simulink model "TP4_1"  (R2016a)
settings: Solver=VariableStepAuto  StartTime=0.0  StopTime=4*pi*sqrt(10/9.81)  FixedStep=4*pi*sqrt(10/9.81) / 500  RelTol=1e-6
undefined symbols (not defined in the file): DiscIntNeverNeededParam, sigbuilder_block
libraries: simulink x5
settings Model: Creator=nsurbayr  LastModifiedBy=nsurbayr
settings DebuggingCC: MultiTaskRateTransMsg=warning

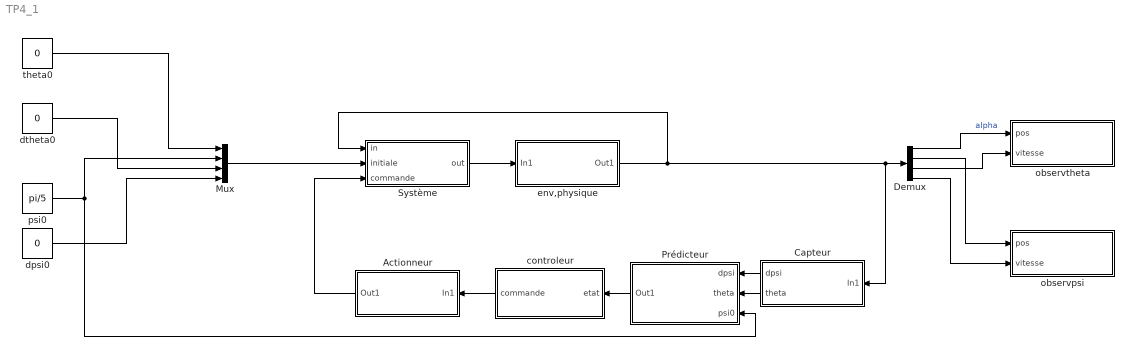
== system TP4_1 ==
  Actionneur : Subsystem
  Capteur : Subsystem
  Demux : Demux
  Mux : Mux
  Prédicteur : Subsystem
  Système : Subsystem
  controleur : Subsystem
  dpsi0 : Constant  Value=0  VectorParams1D=off
  dtheta0 : Constant  Value=0  VectorParams1D=off
  env,physique : Subsystem
  observpsi : Subsystem
  observtheta : Subsystem
  psi0 : Constant  Value=pi/5  VectorParams1D=off
  theta0 : Constant  Value=0
  wires:
  Système/1(out) -> env,physique/1(In1)
  controleur/1(commande) -> Actionneur/1(In1)
  Actionneur/1(Out1) -> Système/3(commande)
  env,physique/1(Out1) -> Système/1(in), Capteur/1(In1), Demux/1
  Prédicteur/1(Out1) -> controleur/1(etat)
  Capteur/1(dpsi) -> Prédicteur/1(dpsi)
  theta0/1 -> Mux/1
  Mux/1 -> Système/2(initiale)
  psi0/1 -> Prédicteur/3("psi0 "), Mux/2
  dtheta0/1 -> Mux/3
  dpsi0/1 -> Mux/4
  Demux/1 -> observtheta/1(pos)  "alpha"
  Demux/2 -> observpsi/1(pos)
  Demux/3 -> observtheta/2(vitesse)
  Demux/4 -> observpsi/2(vitesse)
  Capteur/2(theta) -> Prédicteur/2(theta)

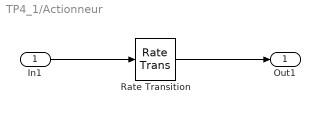
== system TP4_1/Actionneur ==
  In1 : Inport
  Rate Transition : RateTransition  X0=-1
  Out1 : Outport
  wires:
  Rate Transition/1 -> Out1/1
  In1/1 -> Rate Transition/1

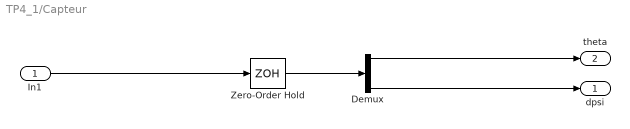
== system TP4_1/Capteur ==
  In1 : Inport
  Demux : Demux
  Zero-Order Hold : ZeroOrderHold  SampleTime=0.003
  dpsi : Outport
  theta : Outport  Port=2
  wires:
  In1/1 -> Zero-Order Hold/1
  Zero-Order Hold/1 -> Demux/1
  Demux/4 -> dpsi/1
  Demux/1 -> theta/1

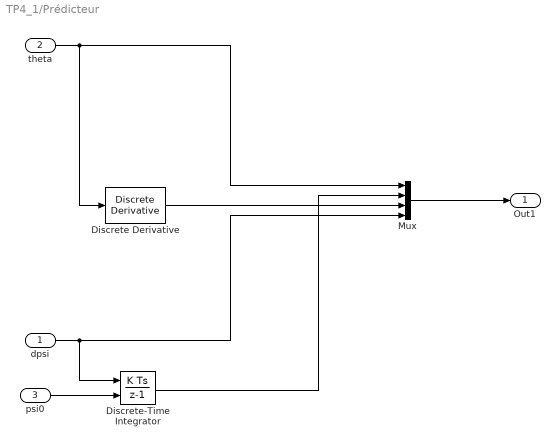
== system TP4_1/Prédicteur ==
  dpsi : Inport
  theta : Inport  Port=2
  "psi0 " : Inport  Port=3
  Discrete Derivative : simulink/Discrete/Discrete Derivative  gainval=1.0  ICPrevScaledInput=0.0  OutMin=[]  OutMax=[]  OutDataType=fixdt(1, 16)  OutScaling=2^-10  DoSatur=off
  Discrete-Time Integrator : DiscreteIntegrator  InitialConditionSource=external  InitialConditionSetting=State (most efficient)  SampleTime=-1  ICPrevOutput=DiscIntNeverNeededParam  ICPrevScaledInput=DiscIntNeverNeededParam
  Mux : Mux
  Out1 : Outport
  wires:
  Mux/1 -> Out1/1
  theta/1 -> Discrete Derivative/1, Mux/1
  dpsi/1 -> Discrete-Time Integrator/1, Mux/4
  Discrete Derivative/1 -> Mux/3
  "psi0 "/1 -> Discrete-Time Integrator/2
  Discrete-Time Integrator/1 -> Mux/2

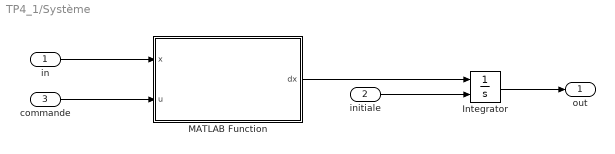
== system TP4_1/Système ==
  in : Inport
  initiale : Inport  Port=2
  commande : Inport  Port=3
  Integrator : Integrator  InitialConditionSource=external
  MATLAB Function : MATLAB Function  TreatAsAtomicUnit=on
      settings: RTWSystemCode=Inline
  out : Outport
  wires:
  Integrator/1 -> out/1
  initiale/1 -> Integrator/2
  in/1 -> MATLAB Function/1(x)
  commande/1 -> MATLAB Function/2(u)
  MATLAB Function/1(dx) -> Integrator/1

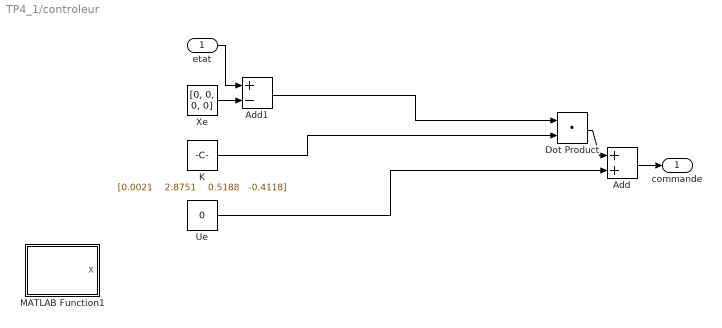
== system TP4_1/controleur ==
  etat : Inport
  Add : Sum
  Add1 : Sum  Inputs=+-
  Dot Product : DotProduct  InputSameDT=on  OutDataTypeStr=Inherit: Inherit via internal rule
  K : Constant  Value="[0.0021    2.8751    0.5188   -0.4118]"
  MATLAB Function1 : MATLAB Function  TreatAsAtomicUnit=on
  Ue : Constant  Value=0
  Xe : Constant  Value=[0, 0, 0, 0]
  commande : Outport
  wires:
  Add/1 -> commande/1
  Ue/1 -> Add/2
  Dot Product/1 -> Add/1
  K/1 -> Dot Product/2
  Xe/1 -> Add1/2
  etat/1 -> Add1/1
  Add1/1 -> Dot Product/1

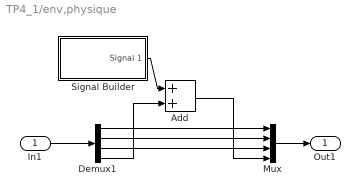
== system TP4_1/env,physique ==
  In1 : Inport
  Add : Sum
  Demux1 : Demux
  Mux : Mux
  Signal Builder : Subsystem  Tag=STV Subsys  LoadFcn=sigbuilder_block('load');  StartFcn=sigbuilder_block('start');  StopFcn=sigbuilder_block('stop');  ClipboardFcn=sigbuilder_block('clipboard');  mask(Sigbuilder block){}
      mask help: Simulink:masks:SigbuilderBlock_MD
      mask init:
      | if ~strcmp(get_param(bdroot(gcbh),'SimulationStatus'),'stopped') tuvar = sigbuilder_block('maskInit'); end
      settings: CopyFcn=sigbuilder_block('copy');  DeleteFcn=sigbuilder_block('delete');  ModelCloseFcn=sigbuilder_block('modelClose');  PreSaveFcn=sigbuilder_block('preSave');  PauseFcn=sigbuilder_block('pause');  ContinueFcn=sigbuilder_block('continue');  NameChangeFcn=sigbuilder_block('namechange');  OpenFcn=sigbuilder_block('open',[416.084 170.526 586.611 354.695 ]);  CloseFcn=sigbuilder_block('close');
      mask Display: plot(0, 0, 100, 100,[2, 2, 32, 32, 2], [68, 8, 8, 68, 68],[32, 2], [38, 38], [32, 19, 2],[53, 60, 44], [32, 17, 17, 2],[16, 16, 31, 31]);txt = getActiveGroup(gcbh);text(2, 100, txt,'verticalAlignment', 'top');
  Out1 : Outport
  wires:
  Demux1/1 -> Mux/1
  Signal Builder/1(Signal 1) -> Add/1
  In1/1 -> Demux1/1
  Mux/1 -> Out1/1
  Demux1/4 -> Add/2
  Add/1 -> Mux/4
  Demux1/2 -> Mux/2
  Demux1/3 -> Mux/3

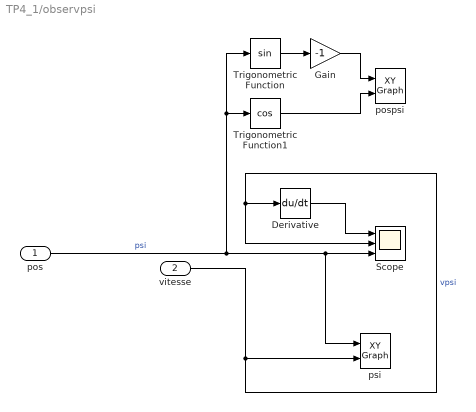
== system TP4_1/observpsi ==
  pos : Inport
  vitesse : Inport  Port=2
  Derivative : Derivative
  Gain : Gain  Gain=-1
  Scope : Scope  NumInputPorts=3
  Trigonometric Function : Trigonometry
  Trigonometric Function1 : Trigonometry  Operator=cos
  pospsi : simulink/Sinks/XY Graph  xmin=-1  xmax=1  ymin=-1  ymax=1  st=-1
  psi : simulink/Sinks/XY Graph  xmin=-pi  xmax=pi  ymin=-2  ymax=2  st=-1
  wires:
  vitesse/1 -> Scope/2, Derivative/1, psi/2  "vpsi"
  pos/1 -> Trigonometric Function/1, Trigonometric Function1/1, Scope/3, psi/1  "psi"
  Derivative/1 -> Scope/1
  Trigonometric Function/1 -> Gain/1
  Gain/1 -> pospsi/1
  Trigonometric Function1/1 -> pospsi/2

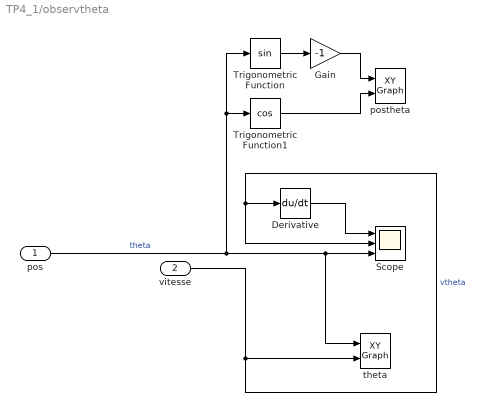
== system TP4_1/observtheta ==
  pos : Inport
  vitesse : Inport  Port=2
  Derivative : Derivative
  Gain : Gain  Gain=-1
  Scope : Scope  NumInputPorts=3
  Trigonometric Function : Trigonometry
  Trigonometric Function1 : Trigonometry  Operator=cos
  postheta : simulink/Sinks/XY Graph  xmin=-1  xmax=1  ymin=-1  ymax=1  st=-1
  theta : simulink/Sinks/XY Graph  xmin=-pi  xmax=pi  ymin=-2  ymax=2  st=-1
  wires:
  vitesse/1 -> Scope/2, Derivative/1, theta/2  "vtheta"
  pos/1 -> Trigonometric Function/1, Trigonometric Function1/1, Scope/3, theta/1  "theta"
  Derivative/1 -> Scope/1
  Trigonometric Function/1 -> Gain/1
  Gain/1 -> postheta/1
  Trigonometric Function1/1 -> postheta/2

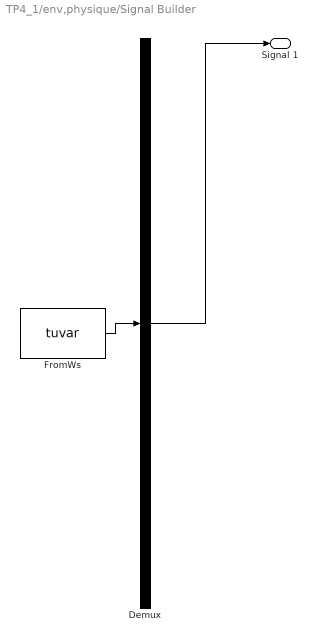
== system TP4_1/env,physique/Signal Builder ==
  Demux : Demux  Tag=STV Demux  Outputs=1
  FromWs : FromWorkspace  Tag=STV FromWs  VariableName=tuvar  SampleTime=0
      SigBuilderData=|
      | common.afterFinalStr = 'Extrapolate'
      | common.sampleTime = 0
      | dataSet.timeRange = [0 20]
      | dataSet.name = 'Group 1'
      | sbobj.Groups.Name = 'Group 1'
      | sbobj.Groups.Signals.Name = 'Signal 1'
      | sbobj.Groups.Signals.XData = [0 6.45 6.45 8.75 8.75 20]
      | sbobj.Groups.Signals.YData = [0 0 2.465 2.465 0 0]
      | sbobj.Groups.TimeRange = [0 20]
  Signal 1 : Outport  Tag=STV Outport
  wires:
  Demux/1 -> Signal 1/1
  FromWs/1 -> Demux/1

== matlab function TP4_1/Système/MATLAB Function ==
  data: x input; u input; dx output
function dx   = fonction( x, u)
%   Dynamic equations of motion of the segway on an axis.
%   Inputs: - x = [theta psi dtheta dpsi]
%               theta: average angle of the wheels      [rad]
%               psi: body pitch angle                   [rad]
%               dtheta: average velocity of the wheels  [rad/s]
%               dpsi: body pitch velocity               [rad/s]
%          - u: DC motor voltage (same value for both motors) [V]

    % State
    psi = x(2);
    dtheta = x(3);
    dpsi = x(4);

    % Parameters
    
    g = 9.81;           % gravity acceleration [m/sec^2]
    m = 0.03;           % wheel weight [kg]
    R = 0.04;           % wheel radius [m]
    Jw = m*R^2/2;       % wheel inertia moment [kg*m^2]
    M = 0.6;            % body weight [kg]
    H = 0.144;          % body height [m]
    L = H/2;            % distance of the center of mass from the wheel axle [m]
    Jpsi = M*L^2/3;     % body pitch inertia [kgm^2]
    Jm = 1e-5;          % DC motor inertia moment [kgm^2]
    Rm = 6.69;          % DC motor resistance [Ohm]
    Kb = 0.468;         % DC motor back EMF constant [Vsec/rad]
    Kt = 0.317;         % DC motor torque constant [Nm/A]
    n = 1;              % gear ratio
    fm = 0.0022;        % friction coefficient between body and DC motor
    fw = 0;             % friction coefficient between wheel and floor
    
    % Equations of motion
    c1 = (2*m+M)*R^2 + 2*Jw + 2*n^2*Jm;
    c2 = M*L*R*cos(psi) - 2*n^2*Jm;
    c3 = -M*L*R*dpsi^2*sin(psi);
    c4 = M*L^2 + Jpsi + 2*n^2*Jm;
    c5 = -M*g*L*sin(psi);

    alpha = Kt/Rm;
    beta = Kt*Kb/Rm + fm;

    Ftheta = alpha*(2*u) - 2*(beta+fw)*dtheta + 2*beta*dpsi;
    Fpsi = -alpha*(2*u) + 2*beta*dtheta - 2*beta*dpsi;

    ddtheta = (c4*c3 - c2*c5 + c4*Ftheta - c2*Fpsi)/(c4*c1 - c2^2);
    ddpsi = (Fpsi- c2*ddtheta - c5)/c4;
    dx = [dtheta dpsi ddtheta ddpsi]';

end

% Matrices of the linearized system
% E = [(2*m+M)*R^2+2*Jw+2*Jm   M*L*R-2*Jm; M*L*R-2*Jm   M*L^2+Jpsi+2*Jm];
% detE = det(E);

% alpha = Kt/Rm;
% beta = Kt*Kb/Rm + fm;

% A32 = -M*g*L*E(1,2)/detE;
% A42 = M*g*L*E(1,1)/detE;
% A33 = -(beta*E(2,2)+2*beta*E(1,2))/detE;
% A43 = (beta*E(1,2)+2*beta*E(1,1))/detE;
% A34 = beta*(E(2,2)+2*E(1,2))/detE;
% A44 = -beta*(E(1,2)+2*E(1,1))/detE;

% B3 = alpha*(E(2,2)/2+E(1,2))/detE;
% B4 = -alpha*(E(1,2)/2+E(1,1))/detE;

% A = [0 0 1 0;0 0 0 1; 0 A32 A33 A34; 0 A42 A43 A44];
% B = [0 0 2*B3 2*B4];

== matlab function TP4_1/controleur/MATLAB Function1 ==
  data: X output
function X = f

% Parameters
    
g = 9.81;           % gravity acceleration [m/sec^2]
m = 0.03;           % wheel weight [kg]
R = 0.04;           % wheel radius [m]
Jw = m*R^2/2;       % wheel inertia moment [kg*m^2]
M = 0.6;            % body weight [kg]
H = 0.144;          % body height [m]
L = H/2;            % distance of the center of mass from the wheel axle [m]
Jpsi = M*L^2/3;     % body pitch inertia [kgm^2]
Jm = 1e-5;          % DC motor inertia moment [kgm^2]
Rm = 6.69;          % DC motor resistance [Ohm]
Kb = 0.468;         % DC motor back EMF constant [Vsec/rad]
Kt = 0.317;         % DC motor torque constant [Nm/A]
n = 1;              % gear ratio
fm = 0.0022;        % friction coefficient between body and DC motor
fw = 0;             % friction coefficient between wheel and floor
    

% Matrices of the linearized system
E = [(2*m+M)*R^2+2*Jw+2*Jm   M*L*R-2*Jm; M*L*R-2*Jm   M*L^2+Jpsi+2*Jm];
detE = det(E);

alpha = Kt/Rm;
beta = Kt*Kb/Rm + fm;

A32 = -M*g*L*E(1,2)/detE;
A42 = M*g*L*E(1,1)/detE;
A33 = -(beta*E(2,2)+2*beta*E(1,2))/detE;
A43 = (beta*E(1,2)+2*beta*E(1,1))/detE;
A34 = beta*(E(2,2)+2*E(1,2))/detE;
A44 = -beta*(E(1,2)+2*E(1,1))/detE;

B3 = alpha*(E(2,2)/2+E(1,2))/detE;
B4 = -alpha*(E(1,2)/2+E(1,1))/detE;

A = [0 0 1 0;0 0 0 1; 0 A32 A33 A34; 0 A42 A43 A44];
B = [0 0 2*B3 2*B4]';
X  = 0;%-place(A,B,[-10,-20,-30,-40])
